simulink model "MaTest"  (R2018b)
settings: Solver=ode45  StartTime=0.0  StopTime=20  MaxStep=1e-3  RelTol=1e-3  AbsTol=1e-4
settings Model: Creator=RUZHOU  LastModifiedBy=RUZHOU

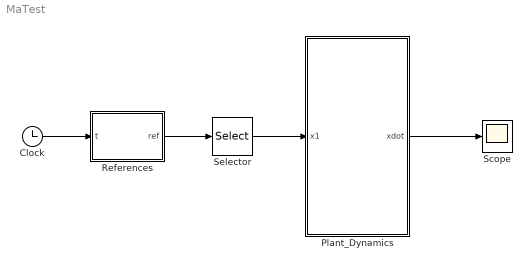
== system MaTest ==
  Clock : Clock
  Plant_Dynamics : MATLAB Function  TreatAsAtomicUnit=on
  References : MATLAB Function  TreatAsAtomicUnit=on
  Scope : Scope
  Selector : Selector  InputPortWidth=8  IndexOptions=Index vector (dialog)  Indices=[1 2]  OutputSizes=1
  wires:
  Clock/1 -> References/1(t)
  References/1(ref) -> Selector/1
  Selector/1 -> Plant_Dynamics/1(x1)
  Plant_Dynamics/1(xdot) -> Scope/1

== matlab function MaTest/Plant_Dynamics ==
  data: x1 input size=2; xdot output
function xdot = fcn(x1)

%% Nonlinear Functions
% Ma
Ma = zeros(2,2);
Ma(1,1) = 2547 + 5400*(sin(x1(2)))^2 - 2*sin(x1(2))*cos(x1(2)) + 224*(cos(x1(2)))^2;
Ma(1,2) = 2.8*sin(x1(2)) + 13.7*cos(x1(2));
Ma(2,1) = Ma(1,2);
Ma(2,2) = 5343;



xdot = eig(Ma);
end

== matlab function MaTest/References ==
  data: t input; ref output size=8
function ref = fcn(t)
% parameters
f1 = 0.1; a1 = 0.5; f2 = 0.15; a2 = 0.2;
x1d = [a1*sin(2*pi*f1*t);a2*sin(2*pi*f2*t)];
x1d_dot = [a1*2*pi*f1*cos(2*pi*f1*t);a2*2*pi*f2*cos(2*pi*f2*t)];
x1d_ddot = [-a1*(2*pi*f1)^2*sin(2*pi*f1*t);-a2*(2*pi*f2)^2*sin(2*pi*f2*t)];
x1d_3dot = [-a1*(2*pi*f1)^3*cos(2*pi*f1*t);-a2*(2*pi*f2)^3*cos(2*pi*f2*t)];
ref = [x1d;x1d_dot;x1d_ddot;x1d_3dot];
end
